simulink model "CURR_SIMULATION"  (R2019b)
settings: Solver=VariableStepAuto  StartTime=0.0  StopTime=100  RelTol=1e-3
undefined symbols (not defined in the file or in its folder): B_friction, Inom, Jm, km, kt, Lm, Rm
libraries: SignalEditorBlockLib x1
settings Model: Creator=peter  LastModifiedBy=peter

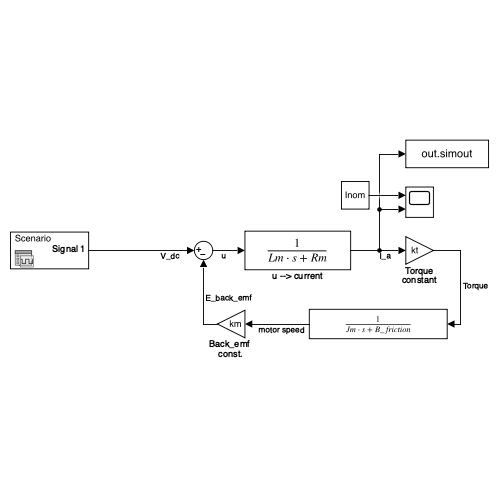
[thumbnail: Simulink's stored preview of the top-level diagram]
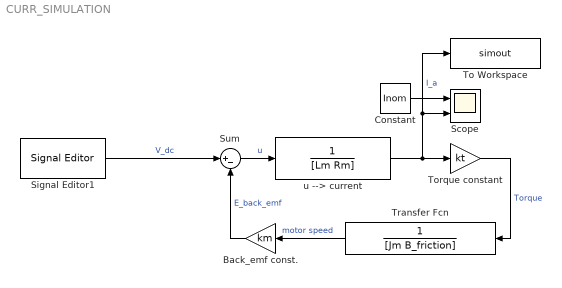
== system CURR_SIMULATION ==
  Back_emf const. : Gain  Gain=km
  Constant : Constant  Value=Inom
  Scope : Scope  NumInputPorts=2
  Signal Editor1 : SignalEditorBlockLib/Signal Editor  FileName=Vdc_TEST.mat  ActiveScenario=Scenario  ActiveSignal=Signal 1  IsBus=off  OutputBusObjectStr=Bus: BusObject  SampleTime=0  Interpolate=off  ZeroCross=off  OutputAfterFinalValue=Setting to zero  Unit=inherit  PreserveSignalName=on
  Sum : Sum  Inputs=|+-
  To Workspace : ToWorkspace  VariableName=simout  SaveFormat=Timeseries  SampleTime=-1
  Torque constant : Gain  Gain=kt
  Transfer Fcn : TransferFcn  Denominator=[Jm B_friction]
  u --> current : TransferFcn  Denominator=[Lm Rm]
  wires:
  Sum/1 -> u --> current/1  "u"
  u --> current/1 -> To Workspace/1, Scope/2, Torque constant/1  "I_a"
  Torque constant/1 -> Transfer Fcn/1  "Torque"
  Transfer Fcn/1 -> Back_emf const./1  "motor speed"
  Back_emf const./1 -> Sum/2  "E_back_emf"
  Signal Editor1/1 -> Sum/1  "V_dc"
  Constant/1 -> Scope/1
